simulink subsystem "AMK_Interface"  (R2020a)
settings: Solver=VariableStepAuto  StartTime=0.0  StopTime=10.0  RelTol=1e-3
undefined symbols (not defined in the file): TMR
settings Model: Creator=Harjot  LastModifiedBy=Harjot

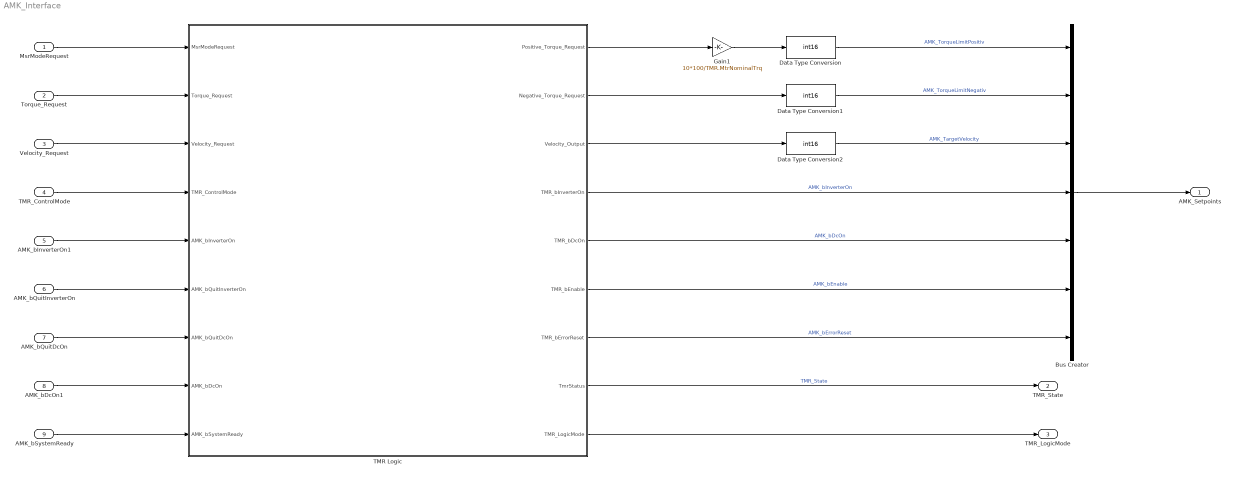
== system AMK_Interface ==
  MsrModeRequest : Inport
  Torque_Request : Inport  Port=2
  Velocity_Request : Inport  Port=3
  TMR_ControlMode : Inport  Port=4
  AMK_bInverterOn1 : Inport  Port=5
  AMK_bQuitInverterOn : Inport  Port=6
  AMK_bQuitDcOn : Inport  Port=7
  AMK_bDcOn1 : Inport  Port=8
  AMK_bSystemReady : Inport  Port=9
  Bus Creator : BusCreator  Inputs=7  OutDataTypeStr=Bus: AmkSetpoints  NonVirtualBus=on
      settings: InheritFromInputs=off
  Data Type Conversion : DataTypeConversion  OutDataTypeStr=int16
  Data Type Conversion1 : DataTypeConversion  OutDataTypeStr=int16
  Data Type Conversion2 : DataTypeConversion  OutDataTypeStr=int16
  Gain1 : Gain  Gain=10*100/TMR.MtrNominalTrq
  TMR Logic : Stateflow chart  TreatAsAtomicUnit=on
  AMK_Setpoints : Outport  OutDataTypeStr=Bus: AmkSetpoints  VectorParamsAs1DForOutWhenUnconnected=off
  TMR_State : Outport  Port=2
  TMR_LogicMode : Outport  Port=3
  wires:
  Velocity_Request/1 -> TMR Logic/3(Velocity_Request)
  TMR Logic/8(TmrStatus) -> TMR_State/1  "TMR_State"
  AMK_bQuitDcOn/1 -> TMR Logic/7(AMK_bQuitDcOn)
  AMK_bQuitInverterOn/1 -> TMR Logic/6(AMK_bQuitInverterOn)
  AMK_bInverterOn1/1 -> TMR Logic/5(AMK_bInverterOn)
  AMK_bDcOn1/1 -> TMR Logic/8(AMK_bDcOn)
  MsrModeRequest/1 -> TMR Logic/1(MsrModeRequest)
  TMR Logic/9(TMR_LogicMode) -> TMR_LogicMode/1
  AMK_bSystemReady/1 -> TMR Logic/9(AMK_bSystemReady)
  TMR_ControlMode/1 -> TMR Logic/4(TMR_ControlMode)
  Torque_Request/1 -> TMR Logic/2(Torque_Request)
  Gain1/1 -> Data Type Conversion/1
  Data Type Conversion/1 -> Bus Creator/1  "AMK_TorqueLimitPositiv"
  Data Type Conversion1/1 -> Bus Creator/2  "AMK_TorqueLimitNegativ"
  Bus Creator/1 -> AMK_Setpoints/1
  Data Type Conversion2/1 -> Bus Creator/3  "AMK_TargetVelocity"
  TMR Logic/1(Positive_Torque_Request) -> Gain1/1
  TMR Logic/2(Negative_Torque_Request) -> Data Type Conversion1/1
  TMR Logic/3(Velocity_Output) -> Data Type Conversion2/1
  TMR Logic/4(TMR_bInverterOn) -> Bus Creator/4  "AMK_bInverterOn"
  TMR Logic/5(TMR_bDcOn) -> Bus Creator/5  "AMK_bDcOn"
  TMR Logic/6(TMR_bEnable) -> Bus Creator/6  "AMK_bEnable"
  TMR Logic/7(TMR_bErrorReset) -> Bus Creator/7  "AMK_bErrorReset"

== stateflow chart AMK_Interface/TMR Logic ==
  state NORMAL_OPERATION
    (history)
    state OFF
      entry:
      TmrStatus = RING_STATUS.OFF;
      Positive_Torque_Request = 0;
      Negative_Torque_Request = 0;
      Velocity_Output = 0;
      TMR_bInverterOn = false;
      TMR_bDcOn = false;
      TMR_bEnable = false;
      TMR_bErrorReset = false;
    state SHUTDOWN
      entry:
      TmrStatus = RING_STATUS.SHUTDOWN_IN_PROGRESS_HV;
      state RequirementsShutDown
        entry:
        Positive_Torque_Request = 0;
        Negative_Torque_Request = 0;
        Velocity_Output = 0;
      state ResetX140BE2
        entry:
        %Reset X140BE2
      state ResetInverterOn
        entry:
        TMR_bInverterOn = false;
      state ResetEnable
        entry:
        TMR_bEnable = false;
      state ResetX140BE1
        entry:
        %Reset X140BE1
      state ShutDown
        entry:
        TmrStatus = RING_STATUS.SHUTDOWN_COMPLETE_HV;
      state CheckQuitDcON1
        entry:
      state ResetX15EF1EF2
        entry:
        %Reset X15EF1/EF2
      state HV_Deactivation
        entry:
        TMR_bDcOn = false;
      (default) -> RequirementsShutDown
      RequirementsShutDown -> ResetX140BE2
      ResetEnable -> ResetX140BE1 : [~AMK_bQuitDcOn]
      ResetX140BE2 -> ResetInverterOn
      ResetInverterOn -> ResetEnable : [~AMK_bInverterOn]
      ResetX140BE1 -> ResetX15EF1EF2
      CheckQuitDcON1 -> ShutDown : [~AMK_bQuitDcOn]
      HV_Deactivation -> CheckQuitDcON1 : [~AMK_bDcOn]
      ResetX15EF1EF2 -> HV_Deactivation
    state OPERATIONAL
      state STARTUP_LV
        entry:
        TmrStatus = RING_STATUS.STARTUP_IN_PROGRESS_LV;
        state AMK_CHECK
          entry:
        state AMK_ONLINE
          entry:
          TmrStatus = RING_STATUS.STARTUP_COMPLETE_LV;
        (default) -> AMK_CHECK
        AMK_CHECK -> AMK_ONLINE : [AMK_bSystemReady]
      state RUNNING
        entry:
        TmrStatus = RING_STATUS.RUNNING;
        state ControlModeOff
          during:
          Positive_Torque_Request = 0;
          Negative_Torque_Request = 0;
          Velocity_Output = 0;
        state SetpointSettingsTorqueControl
          state ForwardAccelSetpointSettingsTorqueControl
            during:
            Velocity_Output = 30000;
            Positive_Torque_Request = Torque_Request;
            Negative_Torque_Request = 0;
          state BrakingSetpointSettingsTorqueControl
            during:
            Velocity_Output = 0; % 750 rpm, = 5km/h
            Positive_Torque_Request = 0;
            Negative_Torque_Request = Torque_Request
          (default) -> (junction 182)
          (junction 182) -> ForwardAccelSetpointSettingsTorqueControl [order 1] : [Torque_Request >= 0]
          (junction 182) -> BrakingSetpointSettingsTorqueControl [order 2]
          ForwardAccelSetpointSettingsTorqueControl -> BrakingSetpointSettingsTorqueControl : [Torque_Request < 0]
          BrakingSetpointSettingsTorqueControl -> ForwardAccelSetpointSettingsTorqueControl : [Torque_Request >= 0]
        state SetpointSettingsSpeedControl
          during:
          Velocity_Output = Velocity_Request;
          Positive_Torque_Request = Torque_Request;
          Negative_Torque_Request = -1*Torque_Request;
        (default) -> ControlModeOff
        ControlModeOff -> SetpointSettingsTorqueControl [order 1] : [TMR_ControlMode == TMR.CONTROL_MODE.TORQUE_CONTROL]
        ControlModeOff -> SetpointSettingsSpeedControl [order 2] : [TMR_ControlMode == TMR.CONTROL_MODE.SPEED_CONTROL]
        SetpointSettingsSpeedControl -> ControlModeOff [order 2] : [TMR_ControlMode == TMR.CONTROL_MODE.OFF]
        SetpointSettingsTorqueControl -> ControlModeOff [order 2] : [TMR_ControlMode == TMR.CONTROL_MODE.OFF]
        SetpointSettingsSpeedControl -> SetpointSettingsTorqueControl [order 1] : [TMR_ControlMode == TMR.CONTROL_MODE.TORQUE_CONTROL]
        SetpointSettingsTorqueControl -> SetpointSettingsSpeedControl [order 1] : [TMR_ControlMode == TMR.CONTROL_MODE.SPEED_CONTROL]
      state STARTUP_HV
        entry:
        TmrStatus = RING_STATUS.STARTUP_IN_PROGRESS_HV;
        state Requirements
          entry:
          Positive_Torque_Request = 0;
          Negative_Torque_Request = 0;
          Velocity_Output = 0;
        state StartingStartUpSequence
        state CheckQuitDcON
          entry:
        state SetX15EF1EF2
          entry:
          %Set X15EF1/EF2
        state HV_Activation
          entry:
          TMR_bDcOn = true;
        state StartUpPass
          entry:
          TmrStatus = RING_STATUS.STARTUP_COMPLETE_HV;
        state SetX140BE2
          entry:
          %Set X140BE2
        state CheckQuitInverterOn
          entry:
        state SetInverterOn
          entry:
          TMR_bInverterOn = true;
        state SetEnable
          entry:
          TMR_bEnable = true;
        state SetX140BE1
          entry:
          %Set X140BE1
        (default) -> StartingStartUpSequence
        Requirements -> SetX15EF1EF2
        CheckQuitDcON -> Requirements : [AMK_bQuitDcOn]
        HV_Activation -> CheckQuitDcON : [AMK_bDcOn]
        StartingStartUpSequence -> HV_Activation
        SetX15EF1EF2 -> SetX140BE1
        SetEnable -> SetInverterOn
        SetX140BE1 -> SetEnable
        SetInverterOn -> CheckQuitInverterOn : [AMK_bInverterOn]
        SetX140BE2 -> StartUpPass
        CheckQuitInverterOn -> SetX140BE2 : [AMK_bQuitInverterOn]
      (default) -> STARTUP_LV
      STARTUP_LV -> STARTUP_HV : [MsrModeRequest == MSR_REQUEST.STARTUP_HV &&...
          |  TmrStatus == RING_STATUS.STARTUP_COMPLETE_LV]
      STARTUP_HV -> RUNNING : [MsrModeRequest == MSR_REQUEST.RUNNING &&...
          | TmrStatus == RING_STATUS.STARTUP_COMPLETE_HV]
    (default) -> OFF
    OPERATIONAL -> SHUTDOWN : [MsrModeRequest == MSR_REQUEST.SHUTDOWN_HV]
    OFF -> OPERATIONAL : [MsrModeRequest == MSR_REQUEST.STARTUP_LV]
  (default) -> NORMAL_OPERATION
  data: MsrModeRequest input Enum: MSR_REQUEST; Torque_Request input; Positive_Torque_Request output double; Negative_Torque_Request output double; Velocity_Output output double; TMR_bInverterOn output boolean; TMR_bDcOn output boolean; TMR_bEnable output boolean; TMR_bErrorReset output boolean; TmrStatus output Enum: RING_STATUS; Velocity_Request input; TMR_ControlMode input; AMK_bInverterOn input boolean; AMK_bQuitInverterOn input boolean; AMK_bQuitDcOn input boolean; AMK_bDcOn input boolean; AMK_bSystemReady input boolean; TMR parameter; TMR_LogicMode output Enum: TMR_LogicModeType
